simulink subsystem "StudentTemplate_M2_draft5"  (R2025a)
settings: Solver=VariableStepAuto  StartTime=0.0  StopTime=10.0  RelTol=1e-3
libraries: slpidlib x7, simulink x5, eeGeneralControl x3
(part 2 of 2)

== stateflow chart StudentTemplate_M2_draft5/encoder_straightening/Chart ==
  state after_turn
    entry:
    during:
    if (LW_dist > RW_dist)
    Right_distance = difference;
    elseif (RW_dist > LW_dist)
    Left_distance =  difference;
    end
  state distance_corrcetion
    exit:
    difference = RW_dist - LW_dist;
    difference = abs(difference)
  (default) -> distance_corrcetion
  after_turn -> distance_corrcetion : [turn_indicator == 1]
  distance_corrcetion -> after_turn : [turn_indicator == 0]
  data: turn_indicator input; RW_dist input; Left_distance output; LW_dist input; Right_distance output; difference local
